simulink model "underwater_gen_2"  (R2021a)
settings: Solver=VariableStepAuto  StartTime=0.0  StopTime=10.0  RelTol=1e-3
libraries: spsACVoltageSourceLib x3, spsDCVoltageSourceLib x2, spsAsynchronousMachineSIUnitsLib x1, spsDCMachineLib x1, spsGroundLib x1, spsSeriesRLCBranchLib x1, spspowerguiLib x1
settings Model: Creator=siddh  LastModifiedBy=siddh

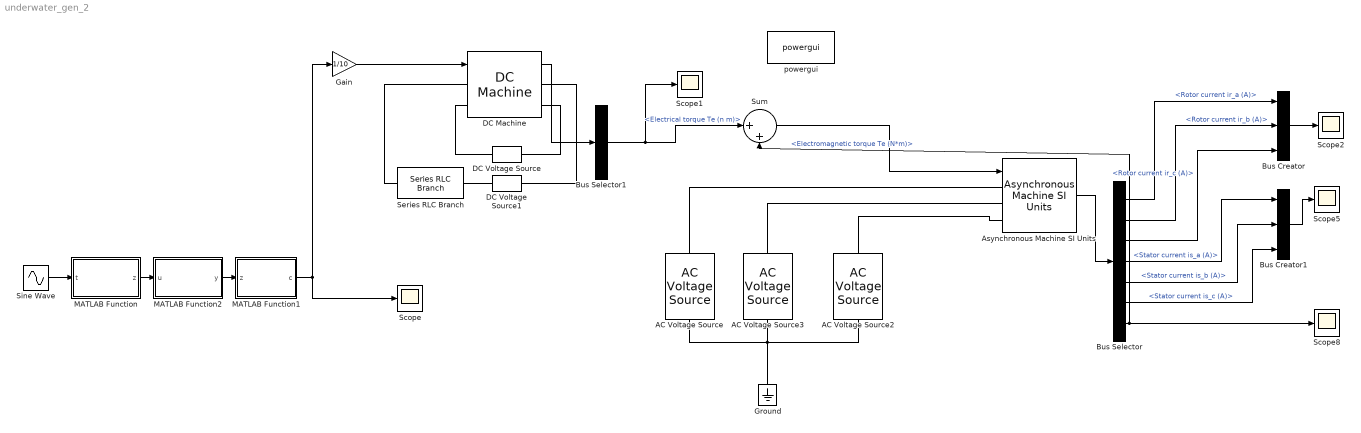
== system underwater_gen_2 ==
  AC Voltage Source : spsACVoltageSourceLib/AC Voltage Source  Amplitude=9000  Phase=0  Frequency=50  SampleTime=0.001  Measurements=None  BusType=swing  Pref=10e3  Qref=0  Qmin=-inf  Qmax=+inf
  AC Voltage Source2 : spsACVoltageSourceLib/AC Voltage Source  Amplitude=9000  Phase=240  Frequency=50  SampleTime=0.001  Measurements=None  BusType=swing  Pref=10e3  Qref=0  Qmin=-inf  Qmax=+inf
  AC Voltage Source3 : spsACVoltageSourceLib/AC Voltage Source  Amplitude=9000  Phase=120  Frequency=50  SampleTime=0.001  Measurements=None  BusType=swing  Pref=10e3  Qref=0  Qmin=-inf  Qmax=+inf
  Asynchronous Machine SI Units : spsAsynchronousMachineSIUnitsLib/Asynchronous Machine SI Units  RotorType=Squirrel-cage  PresetModel=No  MechanicalLoad=Torque Tm  ShowDetailedParameters=on  ReferenceFrame=Rotor  Units=SI  MeasurementBus=off  NominalParameters=[1.845e+04 325.27 50]  VoltageRatio=1  Stator=[0.5968 0.0003495]  Rotor=[0.6258 0.005473]  Cage1=[0.4155 0.002066]  Cage2=[0.4168 0.0003495]  Lm=0.0354  Mechanical=[0.05 0.005879 2]  PolePairs=2  InitialConditions=[0 0 0 0 0 0 0 0]  SimulateSaturation=on  Saturation=[14.03593122, 27.81365428, 53.79336849, 72.68890987, 97.98006896, 148.6815601, 215.7428561, 302.9841135, 428.7778367 ; 230, 322, 414, 460, 506, 552, 598, 644, 690]  LoadFlowParameters=1492000  TsPowergui=0  TsBlock=-1  IterativeModel=Trapezoidal non iterative  IterativeDiscreteModel=Trapezoidal non iterative  Pmec=1.492e+006
  Bus Creator : BusCreator  Inputs=3
  Bus Creator1 : BusCreator  Inputs=3
  Bus Selector : BusSelector  OutputSignals=Rotor measurements.Rotor current ir_a (A),Rotor measurements.Rotor current ir_b (A),Rotor measurements.Rotor current ir_c (A),Stator measurements.Stator current is_a (A),Stator measurements.Stator current is_b (A),Stator measurements.Stator current is_c (A),Mechanical.Electromagnetic torque Te (N*m)
  Bus Selector1 : BusSelector  OutputSignals=Electrical torque Te (n m)
  DC Machine : spsDCMachineLib/DC Machine  PresetModel=No  MechanicalLoad=Speed w  FieldType=Wound  ShowDetailedParameters=on  MeasurementBus=off  RLa="[ 0.6  0.012]"  RLf="[ 240  120]"  Laf=1.8  MachineConstant=Torque constant (N.m/A)  Ke=1.8  Kt=1.8  J=1  Bm=0  Tf=0  w0=1  Ifinit=1.25  TsPowergui=0  TsBlock=-1
  DC Voltage Source : spsDCVoltageSourceLib/DC Voltage Source  Amplitude=300  Measurements=None
  DC Voltage Source1 : spsDCVoltageSourceLib/DC Voltage Source  Amplitude=25.27  Measurements=None
  Gain : Gain  Gain=1/10
  Ground : spsGroundLib/Ground  LConnTagsString=a
  MATLAB Function : MATLAB Function  TreatAsAtomicUnit=on
  MATLAB Function1 : MATLAB Function  TreatAsAtomicUnit=on
  MATLAB Function2 : MATLAB Function  TreatAsAtomicUnit=on
  Scope{,1..2,5,8} (5 alike) : Scope
  Series RLC Branch : spsSeriesRLCBranchLib/Series RLC Branch  LConnTagsString=__new0  RConnTagsString=__new0  BranchType=RLC  Resistance=0.01  Inductance=0  SetiL0=off  InitialCurrent=0  Capacitance=0  Setx0=off  InitialVoltage=0  Measurements=None
  Sine Wave : Sin  Amplitude=4  Frequency=2*pi*1/14  SampleTime=0.001
  Sum : Sum  Inputs=|++
  powergui : spspowerguiLib/powergui  Priority=1  SimulationMode=Continuous  SampleTime=50e-6  frequency=60  Iterations=50  frequencyindice=0  Pbase=100e6  ErrMax=1e-4  UnitsV=kV  UnitsW=MW  buscounter=0  FunctionMessages=off  echomessages=off  EnableUseOfTLC=off  CurrentSourceSwitches=off  DisableSnubberDevices=off  DisableRonSwitches=off  DisableVfSwitches=off  DisplayEquations=off  AutomaticDiscreteSolvers=off  SolverType=Tustin/Backward Euler (TBE)  Interpol=off  ExternalGateDelay=off  methode=off  Ts=100  x0status=blocks  SPID=on  SwTol=0  HookPort=off  NonlinearTolerance=1e-4  nMaxIteration=100  ContinueOnMaxIteration=off  RestoreLinks=warning  ResistiveCurrentMeasurement=off  Frange=[0:2:500]  Ylog=off  Xlog=on  ShowGrid=off  save=off  variable=ZData  structure=0  ZoomFFT=off  StartTime=0.0  cycles=1  DisplayStyle=1  fundamental=60  FreqAxis=off  MaxFrequency=1000  frequencyindicesteady=1  RmsSteady=1  display=off
  wires:
  Asynchronous Machine SI Units/1 -> Bus Selector/1
  Bus Selector/1 -> Bus Creator/1  "<Rotor current ir_a (A)>"
  Bus Selector/2 -> Bus Creator/2  "<Rotor current ir_b (A)>"
  Bus Selector/3 -> Bus Creator/3  "<Rotor current ir_c (A)>"
  Bus Selector/4 -> Bus Creator1/1  "<Stator current is_a (A)>"
  Bus Selector/5 -> Bus Creator1/2  "<Stator current is_b (A)>"
  Bus Selector/6 -> Bus Creator1/3  "<Stator current is_c (A)>"
  Bus Selector/7 -> Sum/2, Scope8/1  "<Electromagnetic torque Te (N*m)>"
  DC Machine/1 -> Bus Selector1/1
  Bus Selector1/1 -> Scope1/1, Sum/1  "<Electrical torque Te (n m)>"
  Sum/1 -> Asynchronous Machine SI Units/1
  Bus Creator/1 -> Scope2/1
  Bus Creator1/1 -> Scope5/1
  MATLAB Function1/1(c) -> Gain/1, Scope/1
  Gain/1 -> DC Machine/1
  Sine Wave/1 -> MATLAB Function/1(t)
  MATLAB Function2/1(y) -> MATLAB Function1/1(z)
  MATLAB Function/1(z) -> MATLAB Function2/1(u)
  connections:
  AC Voltage Source/LConn1 -- Ground/LConn1 -- AC Voltage Source3/LConn1 -- AC Voltage Source2/LConn1
  AC Voltage Source3/RConn1 -- Asynchronous Machine SI Units/LConn2
  AC Voltage Source/RConn1 -- Asynchronous Machine SI Units/LConn1
  AC Voltage Source2/RConn1 -- Asynchronous Machine SI Units/LConn3
  DC Voltage Source/RConn1 -- DC Machine/LConn2
  DC Voltage Source/LConn1 -- DC Machine/RConn2
  Series RLC Branch/RConn1 -- DC Voltage Source1/RConn1
  Series RLC Branch/LConn1 -- DC Machine/LConn1
  DC Voltage Source1/LConn1 -- DC Machine/RConn1

== matlab function underwater_gen_2/MATLAB Function ==
  data: t input; z output
function z = speed_of_waves(t)

z = abs(t);

end

== matlab function underwater_gen_2/MATLAB Function2 ==
  data: u input; y output
function y = Tsunami_protect(u)

if(u>10)
   y = 0;
   
else
    y = u;
end

end

== matlab function underwater_gen_2/MATLAB Function1 ==
  data: z input; c output
function c = clipper(z)

if(z>=4)
   c = 4;

else
    c = z;
end

end
